simulink model "sistema_di_stabilizzazione_meccanico_sm"  (R2023a)
settings: Solver=VariableStepAuto  StartTime=0.0  StopTime=10.0  RelTol=1e-3
settings Model: Creator=giov_russo  LastModifiedBy=miche
settings SolverCC: AlgebraicLoopSolver=TrustRegion
settings DebuggingCC: UnconnectedInputMsg=warning  UnconnectedOutputMsg=warning  UnconnectedLineMsg=warning
settings ModelReferenceCC: EnableRefExpFcnMdlSchedulingChecks=on

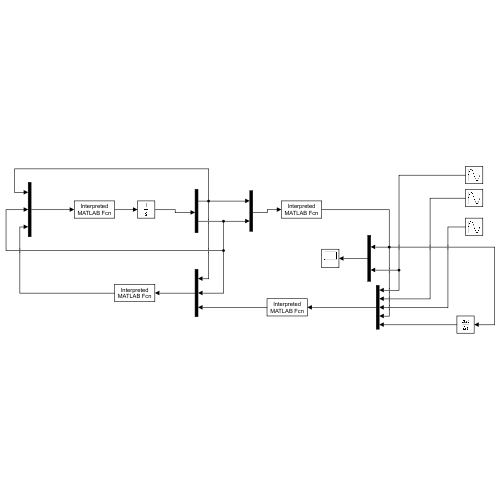
[thumbnail: Simulink's stored preview of the top-level diagram]
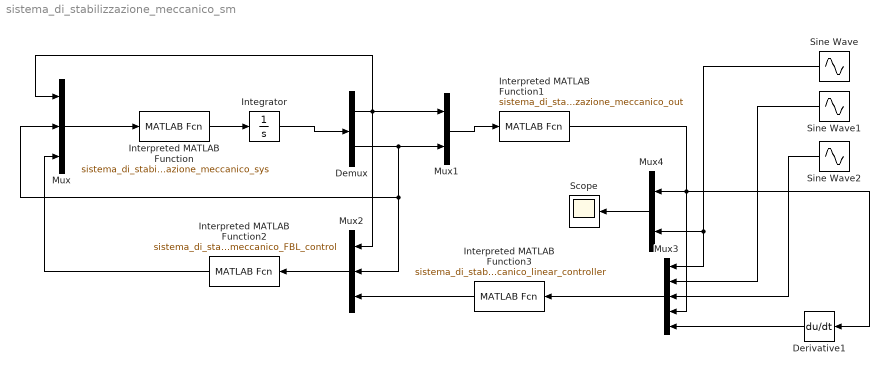
== system sistema_di_stabilizzazione_meccanico_sm ==
  Demux : Demux  Outputs=2
  Derivative1 : Derivative
  Integrator : Integrator
  Interpreted MATLAB Function : MATLABFcn  MATLABFcn=sistema_di_stabilizzazione_meccanico_sys  OutputDimensions=2
  Interpreted MATLAB Function1 : MATLABFcn  MATLABFcn=sistema_di_stabilizzazione_meccanico_out  OutputDimensions=1
  Interpreted MATLAB Function2 : MATLABFcn  MATLABFcn=sistema_di_stabilizzazione_meccanico_FBL_control  OutputDimensions=1
  Interpreted MATLAB Function3 : MATLABFcn  MATLABFcn=sistema_di_stabilizzazione_meccanico_linear_controller  OutputDimensions=1
  Mux : Mux  Inputs=3
  Mux1 : Mux  Inputs=2
  Mux2 : Mux  Inputs=3
  Mux3 : Mux  Inputs=5
  Mux4 : Mux  Inputs=2
  Scope : Scope
  Sine Wave : Sin  SampleTime=0
  Sine Wave1 : Sin  Phase=pi/2  SampleTime=0
  Sine Wave2 : Sin  Amplitude=-1  SampleTime=0
  wires:
  Mux/1 -> Interpreted MATLAB Function/1
  Interpreted MATLAB Function/1 -> Integrator/1
  Integrator/1 -> Demux/1
  Demux/2 -> Mux/2, Mux2/2, Mux1/2
  Mux1/1 -> Interpreted MATLAB Function1/1
  Mux2/1 -> Interpreted MATLAB Function2/1
  Mux3/1 -> Interpreted MATLAB Function3/1
  Mux4/1 -> Scope/1
  Interpreted MATLAB Function2/1 -> Mux/3
  Demux/1 -> Mux/1, Mux1/1, Mux2/1
  Interpreted MATLAB Function3/1 -> Mux2/3
  Sine Wave/1 -> Mux4/2, Mux3/1
  Interpreted MATLAB Function1/1 -> Derivative1/1, Mux3/4, Mux4/1
  Derivative1/1 -> Mux3/5
  Sine Wave1/1 -> Mux3/2
  Sine Wave2/1 -> Mux3/3
